simulink model "OFDM_Tx"  (R2025b)
settings: Solver=FixedStepDiscrete  StartTime=0.0  StopTime=inf  RelTol=1e-3
undefined symbols (not defined in the file): Fs, ip, usb
libraries: hdlsllib x4, commseqgen3 x2, commofdm x2, plutoradiolib x1, commutil2 x1, commdigbbndpm3 x1, commrandsrc3 x1
settings Model: Creator=joann  LastModifiedBy=joann
settings OptimizationCC: OptimizeBlockIOStorage=off  OptimizeDataStoreBuffers=off  BusAssignmentInplaceUpdate=off
settings DebuggingCC: SFUnexpectedBacktrackingDiag=warning  SFNoUnconditionalDefaultTransitionDiag=warning
settings RTWCC: GenerateReport=on  BuildConfiguration=Debug  LaunchReport=on
settings CodeAppCC: ForceParamTrailComments=on  MATLABSourceComments=on  EnableCustomComments=on
settings GRTTargetCC: MultiInstanceErrorCode=Warning  CombineSignalStateStructs=on  SupportVariableSizeSignals=on

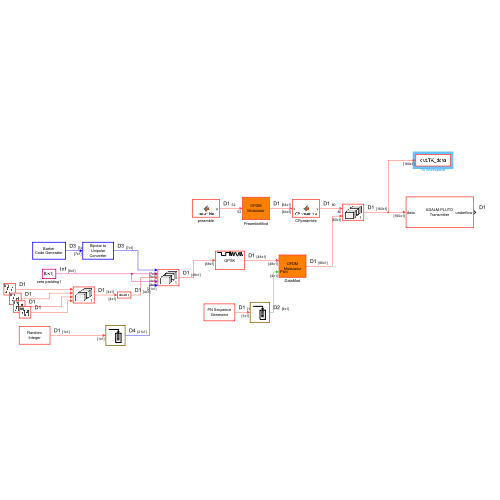
[thumbnail: Simulink's stored preview of the top-level diagram]
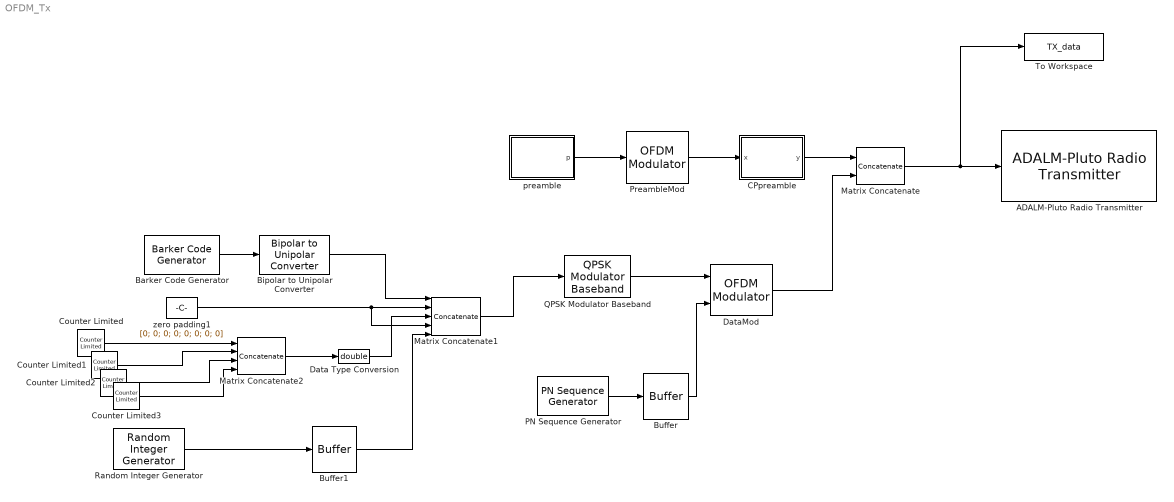
== system OFDM_Tx ==
  ADALM-Pluto Radio Transmitter : plutoradiolib/ADALM-Pluto Radio Transmitter  RadioID=usb:0  uri=ip:10.0.0.200  CenterFrequencySource=Dialog  CenterFrequency=868e6  GainSource=Dialog  Gain=-10  ChannelMapping=1  BasebandSampleRate=100e3  UnderflowOutputPort=on  ShowAdvancedProperties=off  UseCustomFilter=off  filtPathRates=[737280000 11520000 3840000 1920000 960000 240000]  filtCoefficients=[-192 82 85 -215 228 -102 -110 290 -318 145 160 -426 471 -215 -238 633 -697 318 349 -923 1009 -457 -498 1309 -1423 640 693 -1812 1959 -876 -945 2458 -2647 1180 1268 -3290 3534 -1572 -1688 4375 -4698 2091 2247 -5836 6284 -2807 -3031 7918 -8588 3870 4225 -11182 12324 -5662 -6330 17255 -19735 9507 11312 -33568 43355 -25227 -42139 305542 305542 -42139 -25227 43355 -33568 11312 9507 -19735 17255 -6330 -5662 12324 -11182 4225 3870 -8588 7918 -3031 -2807 6284 -5836 2247 2091 -4698 4375 -1688 -1572 3534 -3290 1268 1180 -2647 2458 -945 -876 1959 -1812 693 640 -1423 1309 -498 -457 1009 -923 349 318 -697 633 -238 -215 471 -426 160 145 -318 290 -110 -102 228 -215 85 82 -192]  filtCoefficientSize=128  filtDecimInterpFactor=4  filtGain=-12  filtRFBandwidth=18000000  filterConfigStruct=struct()  DataSourceSelect=Input Port  DDSTone1Freq=5e3  DDSTone2Freq=10e3  DDSTone1Scale=0.5  DDSTone2Scale=0.25  DataTimeout=Inf  FrequencyCorrection=0  ENSMPinControlMode=None  BISTLoopbackMode=Disabled  BISTToneInject=Disabled  BISTSignalGen=PRBS  BISTToneFreq=Fs/32  BISTToneLevel=0
  Barker Code Generator : commseqgen3/Barker Code Generator  Length=7  LengthSimulink=7  SampleTime=1  SamplesPerFrame=7  OutputDataType=double  SimulateUsing=Code generation
  Bipolar to Unipolar Converter : commutil2/Bipolar to Unipolar Converter  M=2  polarity=Positive  dataType=Inherit via internal rule
  Buffer : Buffer  N=4  OutputFrames=off
  Buffer1 : Buffer  N=21  OutputFrames=off
  CPpreamble : MATLAB Function  TreatAsAtomicUnit=on
  Counter Limited{,1..3} (4 alike) : hdlsllib/Sources/Counter Limited  uplimit=3  tsamp=-1
  Data Type Conversion : DataTypeConversion  OutDataTypeStr=double  SaturateOnIntegerOverflow=off  RndMeth=Floor
  DataMod : commofdm/OFDM Modulator  StatePerturbationForJacobian=1.0e-05  FFTLength=64  NumGuardBandCarriers=[6; 5]  InsertDCNull=on  PilotInputPort=on  PilotCarrierIndices=[12; 26; 40; 54]  CyclicPrefixLength=16  Windowing=on  WindowLength=4  OversamplingFactor=1  NumSymbols=1  NumTransmitAntennas=1  SimulateUsing=Interpreted execution
  Matrix Concatenate : Concatenate  Mode=Multidimensional array
  Matrix Concatenate1 : Concatenate  NumInputs=5  Mode=Multidimensional array
  Matrix Concatenate2 : Concatenate  NumInputs=4  Mode=Multidimensional array
  PN Sequence Generator : commseqgen3/PN Sequence Generator  poly='z^8 + z + 1'  ini_sta=[1 0 0 0 1 0 0 1]  outBitMaskSource=Dialog parameter  shift=0  outVarSiz=off  maxOutSizeMode=Dialog parameter  maxOutSize=[10 1]  Ts=1  sampPerFrame=1  reset=off  bitPackedOutputs=off  outDataType=double  numPackedBits=8  bitPackDataSigned=off  bitPackedOutDType=double
      settings: LibrarySourceBlock=|
      | commhdlsource/PN Sequence
      | Generator
  PreambleMod : commofdm/OFDM Modulator  StatePerturbationForJacobian=1.0e-05  FFTLength=64  NumGuardBandCarriers=[6; 5]  InsertDCNull=on  PilotInputPort=off  PilotCarrierIndices=[12; 26; 40; 54]  CyclicPrefixLength=0  Windowing=off  WindowLength=4  OversamplingFactor=1  NumSymbols=1  NumTransmitAntennas=1  SimulateUsing=Code generation
  QPSK Modulator Baseband : commdigbbndpm3/QPSK Modulator Baseband  InType=Integer  Enc=Gray  Ph=pi/4  outDtype=double  outWordLen=16  outUDDataType=sfix(16)  outFracLenMode=Best precision  outFracLen=15  outDataTypeStr=double  outLastDataTypeStr=double
      settings: LibrarySourceBlock=|
      | commhdldigbbndpm/QPSK
      | Modulator
      | Baseband
  Random Integer Generator : commrandsrc3/Random Integer Generator  SetSize=4  SeedSource=Auto  Seed=0  SampleTime=1  SamplesPerFrame=1  OutputDataType=double  SimulateUsing=Interpreted execution
  To Workspace : ToWorkspace  VariableName=TX_data  SaveFormat=Timeseries  SampleTime=-1
  preamble : MATLAB Function  TreatAsAtomicUnit=on
  zero padding1 : Constant  Value=[0; 0; 0; 0; 0; 0; 0; 0]  VectorParams1D=off
  wires:
  preamble/1(p) -> PreambleMod/1
  PreambleMod/1 -> CPpreamble/1(x)
  CPpreamble/1(y) -> Matrix Concatenate/1
  Barker Code Generator/1 -> Bipolar to Unipolar Converter/1
  Bipolar to Unipolar Converter/1 -> Matrix Concatenate1/1
  zero padding1/1 -> Matrix Concatenate1/4, Matrix Concatenate1/2
  Counter Limited/1 -> Matrix Concatenate2/1
  Counter Limited1/1 -> Matrix Concatenate2/2
  Counter Limited2/1 -> Matrix Concatenate2/3
  Counter Limited3/1 -> Matrix Concatenate2/4
  Matrix Concatenate2/1 -> Data Type Conversion/1
  Data Type Conversion/1 -> Matrix Concatenate1/3
  Random Integer Generator/1 -> Buffer1/1
  Matrix Concatenate1/1 -> QPSK Modulator Baseband/1
  QPSK Modulator Baseband/1 -> DataMod/1
  DataMod/1 -> Matrix Concatenate/2
  PN Sequence Generator/1 -> Buffer/1
  Buffer/1 -> DataMod/2
  Matrix Concatenate/1 -> To Workspace/1, ADALM-Pluto Radio Transmitter/1
  Buffer1/1 -> Matrix Concatenate1/5

== matlab function OFDM_Tx/preamble ==
  data: p output
function p = preamble()
%#codegen

% https://dspillustrations.com/pages/posts/misc/schmidlcox-synchronization-for-ofdm.html
% Microsoft Copilot
% https://www.mathworks.com/help/releases/R2025b/comm/ref/pskmod.html


%p = complex( ...
    %[1; 1; -1; -1; 1; -1; -1; 1; 1; -1; 1; 1; -1; 1; 1;...
    %-1; 1; -1; 1; -1; 1; -1; 1; 1; -1; -1; 0;...
    %1; 1; -1; -1; 1; -1; -1; 1; 1; -1; 1; 1; -1; 1; 1;...
    %-1; 1; -1; 1; -1; 1; -1; 1; 1; -1; -1],0);


L = 64; % FFT Length: 64
M = 4; % Modulation Order
numDataSubc = 53; 

% training symbol (used once to get the raw data symbols)
%randomQAM = qammod(randi([0 1], numDataSubc,1),M,true);
%ramdomQAM(2:2:end) = [0];

randomQAM = [-1.0000e+000 +  1.0000e+000i;
     0.0000e+000 +  0.0000e+000i;
    -1.0000e+000 +  1.0000e+000i;
     0.0000e+000 +  0.0000e+000i;
    -1.0000e+000 -  1.0000e+000i;
     0.0000e+000 +  0.0000e+000i;
    -1.0000e+000 +  1.0000e+000i;
     0.0000e+000 +  0.0000e+000i;
    -1.0000e+000 +  1.0000e+000i;
     0.0000e+000 +  0.0000e+000i;
    -1.0000e+000 -  1.0000e+000i;
     0.0000e+000 +  0.0000e+000i;
    -1.0000e+000 -  1.0000e+000i;
     0.0000e+000 +  0.0000e+000i;
    -1.0000e+000 -  1.0000e+000i;
     0.0000e+000 +  0.0000e+000i;
    -1.0000e+000 -  1.0000e+000i;
     0.0000e+000 +  0.0000e+000i;
    -1.0000e+000 +  1.0000e+000i;
     0.0000e+000 +  0.0000e+000i;
    -1.0000e+000 -  1.0000e+000i;
     0.0000e+000 +  0.0000e+000i;
    -1.0000e+000 +  1.0000e+000i;
     0.0000e+000 +  0.0000e+000i;
    -1.0000e+000 +  1.0000e+000i;
     0.0000e+000 +  0.0000e+000i;
    -1.0000e+000 -  1.0000e+000i;
     0.0000e+000 +  0.0000e+000i;
    -1.0000e+000 +  1.0000e+000i;
     0.0000e+000 +  0.0000e+000i;
    -1.0000e+000 -  1.0000e+000i;
     0.0000e+000 +  0.0000e+000i;
    -1.0000e+000 -  1.0000e+000i;
     0.0000e+000 +  0.0000e+000i;
    -1.0000e+000 +  1.0000e+000i;
     0.0000e+000 +  0.0000e+000i;
    -1.0000e+000 -  1.0000e+000i;
     0.0000e+000 +  0.0000e+000i;
    -1.0000e+000 -  1.0000e+000i;
     0.0000e+000 +  0.0000e+000i;
    -1.0000e+000 -  1.0000e+000i;
     0.0000e+000 +  0.0000e+000i;
    -1.0000e+000 -  1.0000e+000i;
     0.0000e+000 +  0.0000e+000i;
    -1.0000e+000 +  1.0000e+000i;
     0.0000e+000 +  0.0000e+000i;
    -1.0000e+000 +  1.0000e+000i;
     0.0000e+000 +  0.0000e+000i;
    -1.0000e+000 -  1.0000e+000i;
     0.0000e+000 +  0.0000e+000i;
    -1.0000e+000 -  1.0000e+000i;
     0.0000e+000 +  0.0000e+000i]; 

p = sqrt(2)*randomQAM;
end

== matlab function OFDM_Tx/CPpreamble ==
  data: y output; x input
function y = CPpreamble(x)
%#codegen

Nfft = 64; % FFT Length (also # of subcarriers)
CP = 16; % Cyclic Prefix Length

half = x(1:Nfft/2);
preambleNoCP = [half;half];
y = [preambleNoCP(end-CP+1:end);preambleNoCP];
end
